simulink model "sldemo_bounce_two_integrators_2018a"  (R2018a)
settings: Solver=ode23  StartTime=0.0  StopTime=20  MaxStep=0.01  RelTol=1e-3  AbsTol=1e-6
libraries: simulink x1
Description:
  | Bouncing Ball Model
  | 
  | This model calculates the trajectory, over time, of a ball thrown
  | upward with a velocity of 15 meters per second from a height of 10 m.
  | The position of the ball is plotted in the upper axis of the scope while
  | the velocity of the ball is plotted in the lower axis. For the
  | recommended approach to modeling a bouncing ball, type
  | 'sldemo_bounce' at the MATLAB prompt.
settings Model: ModifiedByFormat=The MathWorks, Inc.  ExtModeTrigMode=oneshot  ExtModeArmWhenConnect=off  ExtModeAutoUpdateStatusClock=off  Creator=The MathWorks, Inc.  LastModifiedBy=The MathWorks, Inc.
settings SolverCC: AutoScaleAbsTol=off
settings DataIOCC: ExternalInput=[]  InitialState=[]  MaxDataPoints=7500  SaveFormat=Array  SaveOutput=off  DSMLogging=off  SaveTime=off
settings OptimizationCC: BooleanDataType=off  ExpressionDepthLimit=2147483647  InitFltsAndDblsToZero=on  LifeSpan=inf  BufferReusableBoundary=off
settings DebuggingCC: SaveWithParameterizedLinksMsg=none  UnderspecifiedInitializationDetection=Classic  MergeDetectMultiDrivingBlocksExec=none  SignalResolutionControl=TryResolveAllWithWarning  MultiTaskDSMMsg=warning  MultiTaskCondExecSysMsg=none  SigSpecEnsureSampleTimeMsg=none  FcnCallInpInsideContextMsg=warning  BusObjectLabelMismatch=none  StateNameClashWarn=warning  SFUnexpectedBacktrackingDiag=warning  SFNoUnconditionalDefaultTransitionDiag=warning  SFExecutionAtInitializationDiag=none
settings HardwareCC: ProdBitPerPointer=32  ProdBitPerSizeT=32  ProdBitPerPtrDiffT=32  ProdLargestAtomicFloat=None  ProdIntDivRoundTo=Undefined  ProdEndianess=Unspecified  ProdWordSize=32  ProdHWDeviceType=32-bit Generic  TargetBitPerPointer=64  TargetBitPerSizeT=64  TargetBitPerPtrDiffT=64  TargetLongLongMode=on  TargetIntDivRoundTo=Zero  TargetEndianess=LittleEndian  TargetWordSize=64  TargetHWDeviceType=MATLAB Host  ProdEqTarget=off
settings ModelReferenceCC: PropagateSignalLabelsOutOfModel=off
settings RTWCC: Description=Rapid Simulation Target  SystemTargetFile=rsim.tlc  TemplateMakefile=rsim_default_tmf
settings CodeAppCC: StateflowObjectComments=on
settings ConfigComp: CovMetricSettings=d  CovSaveCumulativeToWorkspaceVar=on  CovSaveSingleToWorkspaceVar=on  CovExternalEMLEnable=off

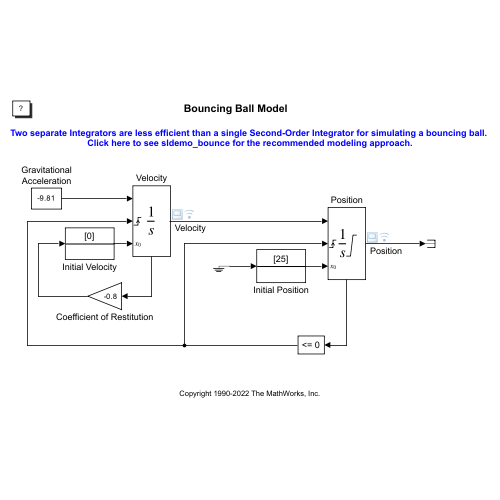
[thumbnail: Simulink's stored preview of the top-level diagram]
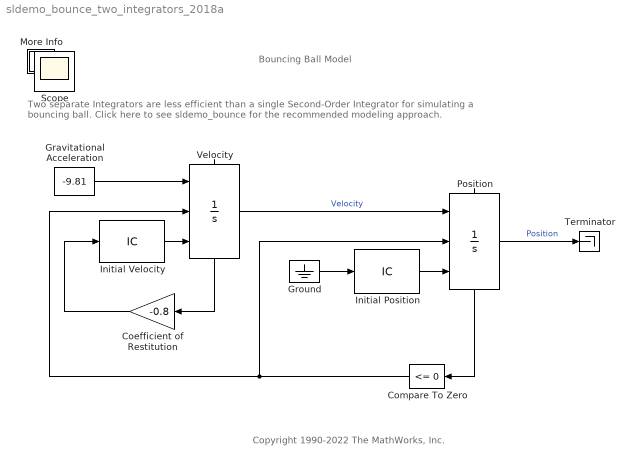
== system sldemo_bounce_two_integrators_2018a ==
  note: Bouncing Ball Model
  note: Two separate Integrators are less efficient than a single Second-Order Integrator for simulating a bouncing ball.
      | Click here to see sldemo_bounce for the recommended modeling approach.
  note: Copyright 1990-2022 The MathWorks, Inc.
  Coefficient of Restitution : Gain  Gain=-0.8  SaturateOnIntegerOverflow=on  OutDataTypeStr=Inherit: Same as input  ParamDataTypeStr=Inherit: Same as input
  Compare To Zero : simulink/Logic and Bit Operations/Compare To Zero  relop=<=  OutDataTypeStr=boolean
  Gravitational Acceleration : Constant  Value=-9.81
  Ground : Ground
  Initial Position : InitialCondition  Value=25
  Initial Velocity : InitialCondition  Value=0
  More Info : Subsystem
      settings: OpenFcn=showExample('simulink_general/sldemo_bounceExample')
      mask Display: disp('?')
  Position : Integrator  ExternalReset=rising  InitialConditionSource=external  LimitOutput=on  LowerSaturationLimit=0  ShowStatePort=on
  Terminator : Terminator
  Velocity : Integrator  ExternalReset=rising  InitialConditionSource=external  ShowStatePort=on
  Scope : Scope
  wires:
  Initial Velocity/1 -> Velocity/3
  Coefficient of Restitution/1 -> Initial Velocity/1
  Velocity/1 -> Position/1  "Velocity"
  Gravitational Acceleration/1 -> Velocity/1
  Ground/1 -> Initial Position/1
  Compare To Zero/1 -> Velocity/2, Position/2
  Initial Position/1 -> Position/3
  Position/1 -> Terminator/1  "Position"
  Position/State -> Compare To Zero/1
  Velocity/State -> Coefficient of Restitution/1

== system sldemo_bounce_two_integrators_2018a/More Info ==
